simulink model "DisertatieVanca"  (R2021b)
settings: Solver=FixedStepAuto  StartTime=0.0  StopTime=10.0  RelTol=1e-3
undefined symbols (not defined in the file): DiscIntNeverNeededParam, Ion, Lithium, Ts, Ts_agent, Ts_speed
libraries: spsSeriesRLCBranchLib x10, spsDiodeLib x7, spsIGBTLib x6, mcbcontrolslib x3, simulink x3, spsVoltageMeasurementLib x3, spsThreePhaseVIMeasurementLib x3, spsCurrentMeasurementLib x2, spsBatteryLib x1, BatteryEstimators x1, spsIGBTDiodeLib x1, slpidlib x1
(part 2 of 2)

== system DisertatieVanca/Errors/BatterySafety ==
  SOC_Battery : Inport
  Voltage_Battery : Inport  Port=2
  Current_Battery : Inport  Port=3
  Power_Bat : Inport  Port=4
  Constant1 : Constant  Value=101  SampleTime=-1
  Constant2 : Constant  Value=-1  SampleTime=-1
  Constant3 : Constant  Value=900  SampleTime=-1
  Constant4 : Constant  Value=0  SampleTime=-1
  Constant6 : Constant  Value=0  SampleTime=-1
  Constant7 : Constant  Value=700  SampleTime=-1
  Constant8 : Constant  Value=0  SampleTime=-1
  Relational Operator1 : RelationalOperator  Operator=>  OutDataTypeStr=boolean  RndMeth=Simplest
  Relational Operator{2,4,6,8} (4 alike) : RelationalOperator  Operator=<  OutDataTypeStr=boolean  RndMeth=Simplest
  Relational Operator3 : RelationalOperator  Operator=>  OutDataTypeStr=boolean  RndMeth=Simplest
  Relational Operator7 : RelationalOperator  Operator=>  OutDataTypeStr=boolean  RndMeth=Simplest
  ErrBatterySOCMallfunctionLow : Outport
  ErrBatterySOCMallfunctionHigh : Outport  Port=2
  ErrBatteryVoltageLow : Outport  Port=3
  ErrBatteryVoltageHigh : Outport  Port=4
  ErrBatteryCurrentLow : Outport  Port=5
  ErrBatteryPowerLow : Outport  Port=6
  ErrBatteryPowerHigh : Outport  Port=7
  wires:
  Relational Operator2/1 -> ErrBatterySOCMallfunctionLow/1
  Relational Operator1/1 -> ErrBatterySOCMallfunctionHigh/1
  SOC_Battery/1 -> Relational Operator2/1, Relational Operator1/1
  Constant1/1 -> Relational Operator1/2
  Voltage_Battery/1 -> Relational Operator4/1, Relational Operator3/1
  Constant3/1 -> Relational Operator3/2
  Relational Operator3/1 -> ErrBatteryVoltageHigh/1
  Relational Operator4/1 -> ErrBatteryVoltageLow/1
  Constant6/1 -> Relational Operator6/1
  Relational Operator6/1 -> ErrBatteryCurrentLow/1
  Current_Battery/1 -> Relational Operator6/2
  Constant7/1 -> Relational Operator7/2
  Power_Bat/1 -> Relational Operator8/1, Relational Operator7/1
  Relational Operator7/1 -> ErrBatteryPowerHigh/1
  Relational Operator8/1 -> ErrBatteryPowerLow/1
  Constant2/1 -> Relational Operator2/2
  Constant4/1 -> Relational Operator4/2
  Constant8/1 -> Relational Operator8/2

== system DisertatieVanca/Errors/DCDCBoostSafety ==
  Vout : Inport
  Vin : Inport  Port=2
  iLref : Inport  Port=3
  Vref : Inport  Port=4
  S : Inport  Port=5
  Constant : Constant  Value=900
  Constant1 : Constant  Value=570  SampleTime=-1
  Constant2 : Constant  Value=480  SampleTime=-1
  Relational Operator : RelationalOperator  OutDataTypeStr=boolean  RndMeth=Simplest
  Relational Operator1 : RelationalOperator  Operator=>  OutDataTypeStr=boolean  RndMeth=Simplest
  Relational Operator2 : RelationalOperator  Operator=<  OutDataTypeStr=boolean  RndMeth=Simplest
  Terminator : Terminator
  Terminator1 : Terminator
  Terminator2 : Terminator
  ErrDCDCBoostOverVoltage : Outport
  ErrDCDCBoostInputVoltageLow : Outport  Port=2
  ErrDCDCBoostInputVoltageHigh : Outport  Port=3
  wires:
  Vout/1 -> Relational Operator/1
  Constant/1 -> Relational Operator/2
  Relational Operator/1 -> ErrDCDCBoostOverVoltage/1
  S/1 -> Terminator/1
  iLref/1 -> Terminator1/1
  Relational Operator1/1 -> ErrDCDCBoostInputVoltageHigh/1
  Constant1/1 -> Relational Operator1/2
  Relational Operator2/1 -> ErrDCDCBoostInputVoltageLow/1
  Vin/1 -> Relational Operator2/1, Relational Operator1/1
  Vref/1 -> Terminator2/1
  Constant2/1 -> Relational Operator2/2

== system DisertatieVanca/Errors/RectifierSafety ==
  VabcTriFazic : Inport
  CurrentValueRectifier : Inport  Port=2
  VoltageRectifier : Inport  Port=3
  MeanVoltageFromRec2 : Inport  Port=4
  MeanVoltageFromRec : Inport  Port=5
  Constant : Constant  Value=350  SampleTime=-1
  Constant1 : Constant  Value=-350  SampleTime=-1
  Constant2 : Constant  Value=700  SampleTime=-1
  Constant3 : Constant  Value=600  SampleTime=-1
  Constant4 : Constant  Value=450  SampleTime=-1
  Relational Operator : RelationalOperator  Operator=>  OutDataTypeStr=boolean  RndMeth=Simplest
  Relational Operator1 : RelationalOperator  Operator=<  OutDataTypeStr=boolean  RndMeth=Simplest
  Relational Operator2 : RelationalOperator  Operator=>  OutDataTypeStr=boolean  RndMeth=Simplest
  Relational Operator3 : RelationalOperator  Operator=>  OutDataTypeStr=boolean  RndMeth=Simplest
  Relational Operator4 : RelationalOperator  Operator=<  OutDataTypeStr=boolean  RndMeth=Simplest
  Terminator : Terminator
  Terminator1 : Terminator
  ErrTriFazicLow : Outport
  ErrTriFazicHigh : Outport  Port=2
  ErrTriFazicOverCurrent : Outport  Port=3
  ErrTriFazicLowVoltage : Outport  Port=4
  ErrTriFazicHighVoltage : Outport  Port=5
  wires:
  VabcTriFazic/1 -> Relational Operator1/1, Relational Operator/1
  Constant/1 -> Relational Operator/2
  Relational Operator/1 -> ErrTriFazicHigh/1
  Relational Operator1/1 -> ErrTriFazicLow/1
  Relational Operator2/1 -> ErrTriFazicOverCurrent/1
  Constant2/1 -> Relational Operator2/2
  CurrentValueRectifier/1 -> Relational Operator2/1
  Relational Operator3/1 -> ErrTriFazicHighVoltage/1
  Constant3/1 -> Relational Operator3/2
  Relational Operator4/1 -> ErrTriFazicLowVoltage/1
  VoltageRectifier/1 -> Relational Operator4/1, Relational Operator3/1
  MeanVoltageFromRec2/1 -> Terminator/1
  MeanVoltageFromRec/1 -> Terminator1/1
  Constant1/1 -> Relational Operator1/2
  Constant4/1 -> Relational Operator4/2

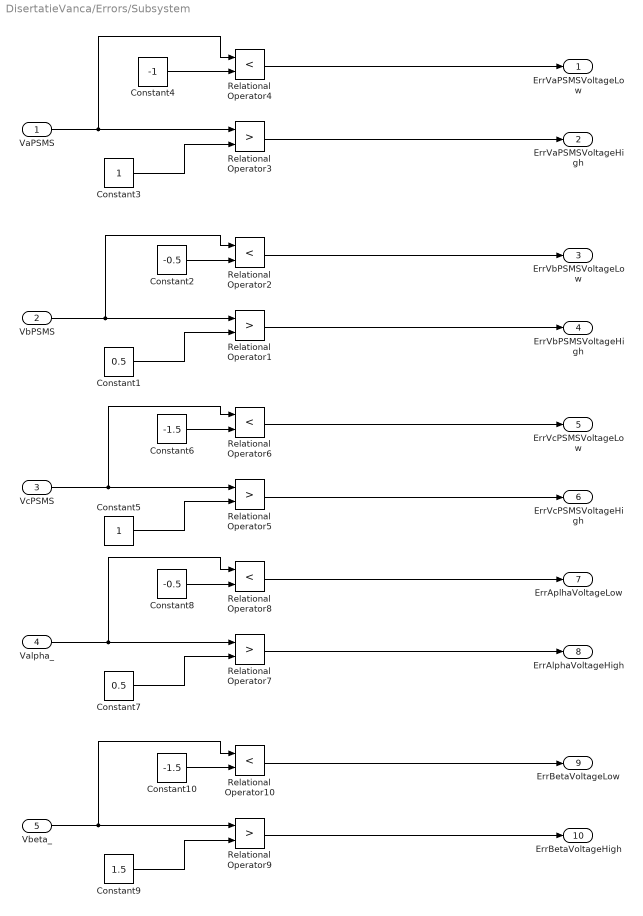
== system DisertatieVanca/Errors/Subsystem ==
  VaPSMS : Inport
  VbPSMS : Inport  Port=2
  VcPSMS : Inport  Port=3
  Valpha_ : Inport  Port=4
  Vbeta_ : Inport  Port=5
  Constant1 : Constant  Value=0.5  SampleTime=-1
  Constant10 : Constant  Value=-1.5  SampleTime=-1
  Constant2 : Constant  Value=-0.5  SampleTime=-1
  Constant3 : Constant  SampleTime=-1
  Constant4 : Constant  Value=-1  SampleTime=-1
  Constant5 : Constant  SampleTime=-1
  Constant6 : Constant  Value=-1.5  SampleTime=-1
  Constant7 : Constant  Value=0.5  SampleTime=-1
  Constant8 : Constant  Value=-0.5  SampleTime=-1
  Constant9 : Constant  Value=1.5  SampleTime=-1
  Relational Operator{1,3,5,7,9} (5 alike) : RelationalOperator  Operator=>  OutDataTypeStr=boolean  RndMeth=Simplest
  Relational Operator{2,4,6,8,10} (5 alike) : RelationalOperator  Operator=<  OutDataTypeStr=boolean  RndMeth=Simplest
  ErrVaPSMSVoltageLow : Outport
  ErrVaPSMSVoltageHigh : Outport  Port=2
  ErrVbPSMSVoltageLow : Outport  Port=3
  ErrVbPSMSVoltageHigh : Outport  Port=4
  ErrVcPSMSVoltageLow : Outport  Port=5
  ErrVcPSMSVoltageHigh : Outport  Port=6
  ErrAplhaVoltageLow : Outport  Port=7
  ErrAlphaVoltageHigh : Outport  Port=8
  ErrBetaVoltageLow : Outport  Port=9
  ErrBetaVoltageHigh : Outport  Port=10
  wires:
  Relational Operator3/1 -> ErrVaPSMSVoltageHigh/1
  Relational Operator4/1 -> ErrVaPSMSVoltageLow/1
  Constant3/1 -> Relational Operator3/2
  VaPSMS/1 -> Relational Operator4/1, Relational Operator3/1
  Relational Operator1/1 -> ErrVbPSMSVoltageHigh/1
  Relational Operator2/1 -> ErrVbPSMSVoltageLow/1
  Constant1/1 -> Relational Operator1/2
  VbPSMS/1 -> Relational Operator2/1, Relational Operator1/1
  Relational Operator5/1 -> ErrVcPSMSVoltageHigh/1
  Relational Operator6/1 -> ErrVcPSMSVoltageLow/1
  Constant5/1 -> Relational Operator5/2
  VcPSMS/1 -> Relational Operator6/1, Relational Operator5/1
  Relational Operator7/1 -> ErrAlphaVoltageHigh/1
  Relational Operator8/1 -> ErrAplhaVoltageLow/1
  Constant7/1 -> Relational Operator7/2
  Valpha_/1 -> Relational Operator8/1, Relational Operator7/1
  Relational Operator9/1 -> ErrBetaVoltageHigh/1
  Relational Operator10/1 -> ErrBetaVoltageLow/1
  Constant9/1 -> Relational Operator9/2
  Vbeta_/1 -> Relational Operator10/1, Relational Operator9/1
  Constant4/1 -> Relational Operator4/2
  Constant2/1 -> Relational Operator2/2
  Constant6/1 -> Relational Operator6/2
  Constant8/1 -> Relational Operator8/2
  Constant10/1 -> Relational Operator10/2

== system DisertatieVanca/Errors/Subsystem1 ==
  IdRef : Inport
  IqRef : Inport  Port=2
  Id_ : Inport  Port=3
  Iq_ : Inport  Port=4
  speed_fb : Inport  Port=5
  speed_ref : Inport  Port=6
  Constant1 : Constant  Value=-1  SampleTime=-1
  Constant10 : Constant  SampleTime=-1
  Constant2 : Constant  SampleTime=-1
  Constant3 : Constant  Value=-1.5  SampleTime=-1
  Constant4 : Constant  Value=1.5  SampleTime=-1
  Constant9 : Constant  Value=3  SampleTime=-1
  Relational Operator1 : RelationalOperator  Operator=<  OutDataTypeStr=boolean  RndMeth=Simplest
  Relational Operator10 : RelationalOperator  Operator=<  OutDataTypeStr=boolean  RndMeth=Simplest
  Relational Operator2 : RelationalOperator  Operator=>  OutDataTypeStr=boolean  RndMeth=Simplest
  Relational Operator3 : RelationalOperator  Operator=<  OutDataTypeStr=boolean  RndMeth=Simplest
  Relational Operator4 : RelationalOperator  Operator=>  OutDataTypeStr=boolean  RndMeth=Simplest
  Relational Operator9 : RelationalOperator  Operator=>  OutDataTypeStr=boolean  RndMeth=Simplest
  Terminator : Terminator
  Terminator1 : Terminator
  Terminator2 : Terminator
  ErrSpeedVoltageLow : Outport
  ErrSpeedVoltageHigh : Outport  Port=2
  ErrIdLow : Outport  Port=3
  ErrIdHigh : Outport  Port=4
  ErrIqLow : Outport  Port=5
  ErrIqHigh : Outport  Port=6
  wires:
  IdRef/1 -> Terminator/1
  IqRef/1 -> Terminator1/1
  speed_ref/1 -> Terminator2/1
  Relational Operator10/1 -> ErrSpeedVoltageLow/1
  Constant9/1 -> Relational Operator9/2
  speed_fb/1 -> Relational Operator10/1, Relational Operator9/1
  Relational Operator9/1 -> ErrSpeedVoltageHigh/1
  Relational Operator1/1 -> ErrIdLow/1
  Constant2/1 -> Relational Operator2/2
  Id_/1 -> Relational Operator1/1, Relational Operator2/1
  Relational Operator2/1 -> ErrIdHigh/1
  Relational Operator3/1 -> ErrIqLow/1
  Constant4/1 -> Relational Operator4/2
  Iq_/1 -> Relational Operator3/1, Relational Operator4/1
  Relational Operator4/1 -> ErrIqHigh/1
  Constant10/1 -> Relational Operator10/2
  Constant1/1 -> Relational Operator1/2
  Constant3/1 -> Relational Operator3/2

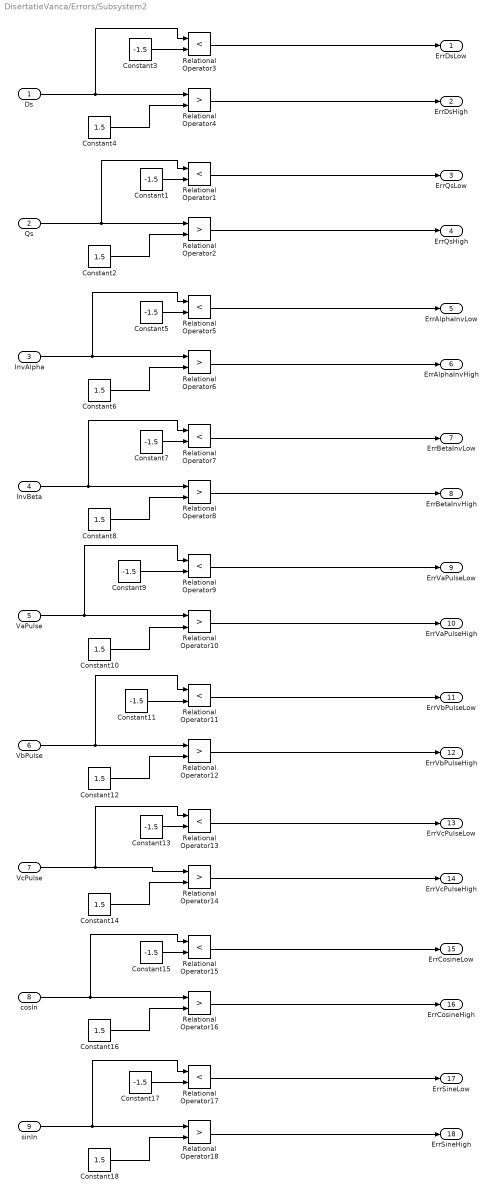
== system DisertatieVanca/Errors/Subsystem2 ==
  Ds : Inport
  Qs : Inport  Port=2
  InvAlpha : Inport  Port=3
  InvBeta : Inport  Port=4
  VaPulse : Inport  Port=5
  VbPulse : Inport  Port=6
  VcPulse : Inport  Port=7
  cosIn : Inport  Port=8
  sinIn : Inport  Port=9
  Constant{1,3,5,7,9,11,13,15,17} (9 alike) : Constant  Value=-1.5  SampleTime=-1
  Constant{2,4,6,8,10,12,14,16,18} (9 alike) : Constant  Value=1.5  SampleTime=-1
  Relational Operator{1,3,5,7,9,11,13,15,17} (9 alike) : RelationalOperator  Operator=<  OutDataTypeStr=boolean  RndMeth=Simplest
  Relational Operator{2,4,6,8,10,12,14,16,18} (9 alike) : RelationalOperator  Operator=>  OutDataTypeStr=boolean  RndMeth=Simplest
  ErrDsLow : Outport
  ErrDsHigh : Outport  Port=2
  ErrQsLow : Outport  Port=3
  ErrQsHigh : Outport  Port=4
  ErrAlphaInvLow : Outport  Port=5
  ErrAlphaInvHigh : Outport  Port=6
  ErrBetaInvLow : Outport  Port=7
  ErrBetaInvHigh : Outport  Port=8
  ErrVaPulseLow : Outport  Port=9
  ErrVaPulseHigh : Outport  Port=10
  ErrVbPulseLow : Outport  Port=11
  ErrVbPulseHigh : Outport  Port=12
  ErrVcPulseLow : Outport  Port=13
  ErrVcPulseHigh : Outport  Port=14
  ErrCosineLow : Outport  Port=15
  ErrCosineHigh : Outport  Port=16
  ErrSineLow : Outport  Port=17
  ErrSineHigh : Outport  Port=18
  wires:
  Relational Operator3/1 -> ErrDsLow/1
  Relational Operator4/1 -> ErrDsHigh/1
  Constant4/1 -> Relational Operator4/2
  Ds/1 -> Relational Operator3/1, Relational Operator4/1
  Relational Operator1/1 -> ErrQsLow/1
  Relational Operator2/1 -> ErrQsHigh/1
  Constant2/1 -> Relational Operator2/2
  Qs/1 -> Relational Operator1/1, Relational Operator2/1
  Relational Operator6/1 -> ErrAlphaInvHigh/1
  Relational Operator5/1 -> ErrAlphaInvLow/1
  InvAlpha/1 -> Relational Operator5/1, Relational Operator6/1
  Constant6/1 -> Relational Operator6/2
  Relational Operator8/1 -> ErrBetaInvHigh/1
  Relational Operator7/1 -> ErrBetaInvLow/1
  InvBeta/1 -> Relational Operator7/1, Relational Operator8/1
  Constant8/1 -> Relational Operator8/2
  VaPulse/1 -> Relational Operator9/1, Relational Operator10/1
  Relational Operator10/1 -> ErrVaPulseHigh/1
  Constant10/1 -> Relational Operator10/2
  Relational Operator9/1 -> ErrVaPulseLow/1
  VbPulse/1 -> Relational Operator11/1, Relational Operator12/1
  Relational Operator12/1 -> ErrVbPulseHigh/1
  Constant12/1 -> Relational Operator12/2
  Relational Operator11/1 -> ErrVbPulseLow/1
  VcPulse/1 -> Relational Operator13/1, Relational Operator14/1
  Relational Operator14/1 -> ErrVcPulseHigh/1
  Constant14/1 -> Relational Operator14/2
  Relational Operator13/1 -> ErrVcPulseLow/1
  cosIn/1 -> Relational Operator15/1, Relational Operator16/1
  Relational Operator16/1 -> ErrCosineHigh/1
  Constant16/1 -> Relational Operator16/2
  Relational Operator15/1 -> ErrCosineLow/1
  sinIn/1 -> Relational Operator17/1, Relational Operator18/1
  Relational Operator18/1 -> ErrSineHigh/1
  Constant18/1 -> Relational Operator18/2
  Relational Operator17/1 -> ErrSineLow/1
  Constant3/1 -> Relational Operator3/2
  Constant1/1 -> Relational Operator1/2
  Constant5/1 -> Relational Operator5/2
  Constant7/1 -> Relational Operator7/2
  Constant9/1 -> Relational Operator9/2
  Constant11/1 -> Relational Operator11/2
  Constant13/1 -> Relational Operator13/2
  Constant15/1 -> Relational Operator15/2
  Constant17/1 -> Relational Operator17/2

== system DisertatieVanca/Errors Clasification/High Severity ==
  ErrTriFazicOverCurrent : Inport
  ErrBatterySOCMallfunctionLow : Inport  Port=2
  ErrBatterySOCMallfunctionHigh : Inport  Port=3
  ErrDCDCBoostOverVoltage : Inport  Port=4
  ErrDCDCBoostInputVoltageHigh : Inport  Port=5
  Bus Creator : BusCreator  Inputs=5
  Constant{,1..4} (5 alike) : Constant  Value=0  SampleTime=-1
  Relational Operator{,1..4} (5 alike) : RelationalOperator  Operator=>  OutDataTypeStr=boolean  RndMeth=Simplest
  High_Severity : Outport
  wires:
  Constant/1 -> Relational Operator/2
  ErrBatterySOCMallfunctionLow/1 -> Relational Operator1/1
  Constant1/1 -> Relational Operator1/2
  ErrBatterySOCMallfunctionHigh/1 -> Relational Operator2/1
  Constant2/1 -> Relational Operator2/2
  ErrDCDCBoostOverVoltage/1 -> Relational Operator3/1
  Constant3/1 -> Relational Operator3/2
  ErrDCDCBoostInputVoltageHigh/1 -> Relational Operator4/1
  Constant4/1 -> Relational Operator4/2
  ErrTriFazicOverCurrent/1 -> Relational Operator/1
  Relational Operator2/1 -> Bus Creator/3
  Relational Operator1/1 -> Bus Creator/2
  Relational Operator/1 -> Bus Creator/1
  Relational Operator3/1 -> Bus Creator/4
  Relational Operator4/1 -> Bus Creator/5
  Bus Creator/1 -> High_Severity/1

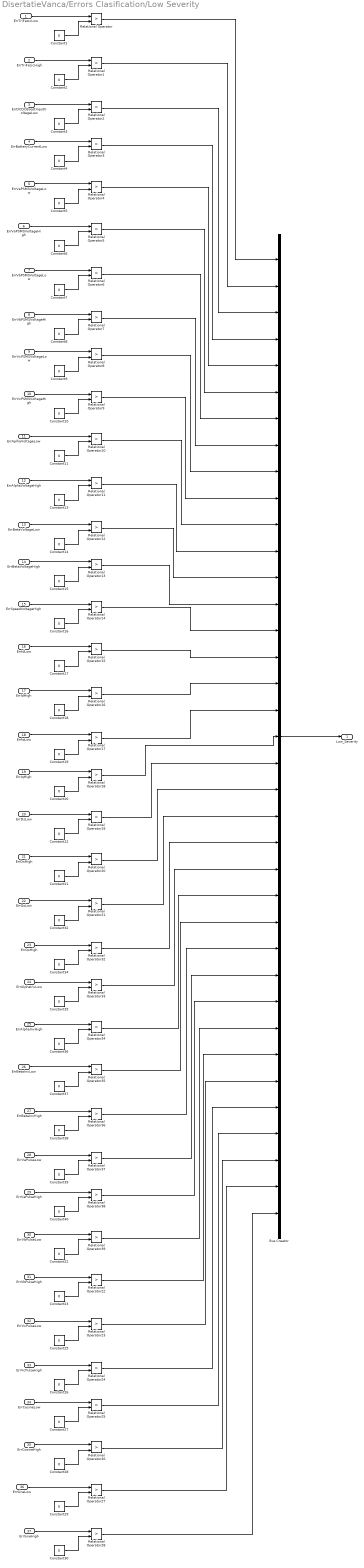
== system DisertatieVanca/Errors Clasification/Low Severity ==
  ErrTriFazicLow : Inport
  ErrTriFazicHigh : Inport  Port=2
  ErrDCDCBoostInputVoltageLow : Inport  Port=3
  ErrBatteryCurrentLow : Inport  Port=4
  ErrVaPSMSVoltageLow : Inport  Port=5
  ErrVaPSMSVoltageHigh : Inport  Port=6
  ErrVbPSMSVoltageLow : Inport  Port=7
  ErrVbPSMSVoltageHigh : Inport  Port=8
  ErrVcPSMSVoltageLow : Inport  Port=9
  ErrVcPSMSVoltageHigh : Inport  Port=10
  ErrAplhaVoltageLow : Inport  Port=11
  ErrAlphaVoltageHigh : Inport  Port=12
  ErrBetaVoltageLow : Inport  Port=13
  ErrBetaVoltageHigh : Inport  Port=14
  ErrSpeedVoltageHigh : Inport  Port=15
  ErrIdLow : Inport  Port=16
  ErrIdHigh : Inport  Port=17
  ErrIqLow : Inport  Port=18
  ErrIqHigh : Inport  Port=19
  ErrDsLow : Inport  Port=20
  ErrDsHigh : Inport  Port=21
  ErrQsLow : Inport  Port=22
  ErrQsHigh : Inport  Port=23
  ErrAlphaInvLow : Inport  Port=24
  ErrAlphaInvHigh : Inport  Port=25
  ErrBetaInvLow : Inport  Port=26
  ErrBetaInvHigh : Inport  Port=27
  ErrVaPulseLow : Inport  Port=28
  ErrVaPulseHigh : Inport  Port=29
  ErrVbPulseLow : Inport  Port=30
  ErrVbPulseHigh : Inport  Port=31
  ErrVcPulseLow : Inport  Port=32
  ErrVcPulseHigh : Inport  Port=33
  ErrCosineLow : Inport  Port=34
  ErrCosineHigh : Inport  Port=35
  ErrSineLow : Inport  Port=36
  ErrSineHigh : Inport  Port=37
  Bus Creator : BusCreator  Inputs=37
  Constant{1..23,25..30,32,34..40} (37 alike) : Constant  Value=0  SampleTime=-1
  Relational Operator{,1..28,32..39} (37 alike) : RelationalOperator  Operator=>  OutDataTypeStr=boolean  RndMeth=Simplest
  Low_Severity : Outport
  wires:
  Constant1/1 -> Relational Operator/2
  ErrTriFazicLow/1 -> Relational Operator/1
  Constant2/1 -> Relational Operator1/2
  ErrTriFazicHigh/1 -> Relational Operator1/1
  Constant3/1 -> Relational Operator2/2
  ErrDCDCBoostInputVoltageLow/1 -> Relational Operator2/1
  Constant4/1 -> Relational Operator3/2
  ErrBatteryCurrentLow/1 -> Relational Operator3/1
  Constant5/1 -> Relational Operator4/2
  ErrVaPSMSVoltageLow/1 -> Relational Operator4/1
  ErrVcPSMSVoltageLow/1 -> Relational Operator8/1
  ErrVaPSMSVoltageHigh/1 -> Relational Operator5/1
  ErrVbPSMSVoltageLow/1 -> Relational Operator6/1
  Constant8/1 -> Relational Operator7/2
  ErrVbPSMSVoltageHigh/1 -> Relational Operator7/1
  ErrVcPSMSVoltageHigh/1 -> Relational Operator9/1
  Constant6/1 -> Relational Operator5/2
  Constant7/1 -> Relational Operator6/2
  Constant10/1 -> Relational Operator9/2
  Constant9/1 -> Relational Operator8/2
  ErrDsLow/1 -> Relational Operator19/1
  ErrBetaVoltageHigh/1 -> Relational Operator13/1
  ErrAplhaVoltageLow/1 -> Relational Operator10/1
  ErrAlphaVoltageHigh/1 -> Relational Operator11/1
  Constant11/1 -> Relational Operator10/2
  ErrSpeedVoltageHigh/1 -> Relational Operator14/1
  Constant15/1 -> Relational Operator13/2
  Constant14/1 -> Relational Operator12/2
  ErrIqLow/1 -> Relational Operator17/1
  ErrIdLow/1 -> Relational Operator15/1
  ErrBetaVoltageLow/1 -> Relational Operator12/1
  Constant20/1 -> Relational Operator18/2
  Constant17/1 -> Relational Operator15/2
  Constant19/1 -> Relational Operator17/2
  Constant18/1 -> Relational Operator16/2
  ErrIqHigh/1 -> Relational Operator18/1
  Constant13/1 -> Relational Operator11/2
  ErrIdHigh/1 -> Relational Operator16/1
  Constant16/1 -> Relational Operator14/2
  Constant12/1 -> Relational Operator19/2
  ErrAlphaInvLow/1 -> Relational Operator33/1
  ErrDsHigh/1 -> Relational Operator20/1
  ErrCosineLow/1 -> Relational Operator25/1
  ErrQsLow/1 -> Relational Operator21/1
  ErrVbPulseHigh/1 -> Relational Operator22/1
  ErrSineHigh/1 -> Relational Operator28/1
  Constant21/1 -> Relational Operator20/2
  ErrAlphaInvHigh/1 -> Relational Operator34/1
  ErrCosineHigh/1 -> Relational Operator26/1
  Constant34/1 -> Relational Operator32/2
  ErrVaPulseLow/1 -> Relational Operator37/1
  ErrSineLow/1 -> Relational Operator27/1
  ErrQsHigh/1 -> Relational Operator32/1
  ErrVcPulseHigh/1 -> Relational Operator24/1
  Constant40/1 -> Relational Operator38/2
  Constant39/1 -> Relational Operator37/2
  Constant37/1 -> Relational Operator35/2
  Constant38/1 -> Relational Operator36/2
  Constant32/1 -> Relational Operator21/2
  Constant30/1 -> Relational Operator28/2
  Constant25/1 -> Relational Operator23/2
  Constant22/1 -> Relational Operator39/2
  Constant27/1 -> Relational Operator25/2
  Constant29/1 -> Relational Operator27/2
  Constant23/1 -> Relational Operator22/2
  ErrVbPulseLow/1 -> Relational Operator39/1
  ErrVaPulseHigh/1 -> Relational Operator38/1
  ErrBetaInvHigh/1 -> Relational Operator36/1
  Constant36/1 -> Relational Operator34/2
  Constant26/1 -> Relational Operator24/2
  Constant35/1 -> Relational Operator33/2
  ErrVcPulseLow/1 -> Relational Operator23/1
  Constant28/1 -> Relational Operator26/2
  ErrBetaInvLow/1 -> Relational Operator35/1
  Relational Operator/1 -> Bus Creator/1
  Relational Operator1/1 -> Bus Creator/2
  Relational Operator2/1 -> Bus Creator/3
  Relational Operator3/1 -> Bus Creator/4
  Relational Operator4/1 -> Bus Creator/5
  Relational Operator5/1 -> Bus Creator/6
  Relational Operator6/1 -> Bus Creator/7
  Relational Operator7/1 -> Bus Creator/8
  Relational Operator8/1 -> Bus Creator/9
  Relational Operator9/1 -> Bus Creator/10
  Relational Operator10/1 -> Bus Creator/11
  Relational Operator11/1 -> Bus Creator/12
  Relational Operator12/1 -> Bus Creator/13
  Relational Operator13/1 -> Bus Creator/14
  Relational Operator14/1 -> Bus Creator/15
  Relational Operator15/1 -> Bus Creator/16
  Relational Operator16/1 -> Bus Creator/17
  Relational Operator17/1 -> Bus Creator/18
  Relational Operator18/1 -> Bus Creator/19
  Relational Operator19/1 -> Bus Creator/20
  Relational Operator20/1 -> Bus Creator/21
  Relational Operator21/1 -> Bus Creator/22
  Relational Operator32/1 -> Bus Creator/23
  Relational Operator33/1 -> Bus Creator/24
  Relational Operator34/1 -> Bus Creator/25
  Relational Operator35/1 -> Bus Creator/26
  Relational Operator36/1 -> Bus Creator/27
  Relational Operator37/1 -> Bus Creator/28
  Relational Operator38/1 -> Bus Creator/29
  Relational Operator39/1 -> Bus Creator/30
  Relational Operator22/1 -> Bus Creator/31
  Relational Operator23/1 -> Bus Creator/32
  Relational Operator24/1 -> Bus Creator/33
  Relational Operator25/1 -> Bus Creator/34
  Relational Operator26/1 -> Bus Creator/35
  Relational Operator27/1 -> Bus Creator/36
  Relational Operator28/1 -> Bus Creator/37
  Bus Creator/1 -> Low_Severity/1

== system DisertatieVanca/Errors Clasification/Medium Severity ==
  ErrTriFazicLowVoltage : Inport
  ErrTriFazicHighVoltage : Inport  Port=2
  ErrBatteryVoltageLow : Inport  Port=3
  ErrBatteryVoltageHigh : Inport  Port=4
  ErrBatteryPowerLow : Inport  Port=5
  ErrBatteryPowerHigh : Inport  Port=6
  ErrSpeedVoltageLow : Inport  Port=7
  Bus Creator : BusCreator  Inputs=7
  Constant{1..7} (7 alike) : Constant  Value=0  SampleTime=-1
  Relational Operator{,1..6} (7 alike) : RelationalOperator  Operator=>  OutDataTypeStr=boolean  RndMeth=Simplest
  Medium_Severity : Outport
  wires:
  ErrTriFazicLowVoltage/1 -> Relational Operator/1
  Constant1/1 -> Relational Operator/2
  Constant2/1 -> Relational Operator1/2
  ErrTriFazicHighVoltage/1 -> Relational Operator1/1
  Constant3/1 -> Relational Operator2/2
  ErrBatteryVoltageLow/1 -> Relational Operator2/1
  Constant4/1 -> Relational Operator3/2
  ErrBatteryVoltageHigh/1 -> Relational Operator3/1
  Constant5/1 -> Relational Operator4/2
  ErrBatteryPowerLow/1 -> Relational Operator4/1
  Constant6/1 -> Relational Operator5/2
  ErrBatteryPowerHigh/1 -> Relational Operator5/1
  Constant7/1 -> Relational Operator6/2
  ErrSpeedVoltageLow/1 -> Relational Operator6/1
  Relational Operator3/1 -> Bus Creator/4
  Relational Operator2/1 -> Bus Creator/3
  Relational Operator1/1 -> Bus Creator/2
  Relational Operator/1 -> Bus Creator/1
  Relational Operator4/1 -> Bus Creator/5
  Relational Operator5/1 -> Bus Creator/6
  Relational Operator6/1 -> Bus Creator/7
  Bus Creator/1 -> Medium_Severity/1

== system DisertatieVanca/Reinforcement Learning/IsDone ==
  Iq_ref : Inport
  Compare To Constant2 : simulink/Logic and Bit Operations/Compare To Constant  relop=>=  const=0.3  OutDataTypeStr=boolean
  Compare To Constant3 : simulink/Logic and Bit Operations/Compare To Constant  relop=>=  const=1  OutDataTypeStr=boolean
  Digital Clock : DigitalClock  SampleTime=Ts_agent
  OR1 : Logic  IconShape=distinctive  AllPortsSameDT=off  OutDataTypeStr=boolean
  Product : Product
  TrainFlag : Constant  OutDataTypeStr=double
  stop : Outport
  wires:
  TrainFlag/1 -> Product/2
  Product/1 -> stop/1
  Digital Clock/1 -> Compare To Constant2/1
  OR1/1 -> Product/1
  Compare To Constant3/1 -> OR1/1
  Iq_ref/1 -> Compare To Constant3/1
  Compare To Constant2/1 -> OR1/2

== system DisertatieVanca/Reinforcement Learning/Observations ==
  speed ref : Inport
  speed fb : Inport  Port=2
  id err : Inport  Port=3
  id : Inport  Port=4
  iq err : Inport  Port=5
  iq : Inport  Port=6
  Discrete-Time Integrator : DiscreteIntegrator  SampleTime=-1  ICPrevOutput=DiscIntNeverNeededParam  ICPrevScaledInput=DiscIntNeverNeededParam
  Discrete-Time Integrator1 : DiscreteIntegrator  SampleTime=-1  ICPrevOutput=DiscIntNeverNeededParam  ICPrevScaledInput=DiscIntNeverNeededParam
  Mux1 : Mux  Inputs=8
  observations : Outport  VectorParamsAs1DForOutWhenUnconnected=off
  wires:
  id err/1 -> Discrete-Time Integrator/1, Mux1/5
  Discrete-Time Integrator/1 -> Mux1/6
  iq err/1 -> Discrete-Time Integrator1/1, Mux1/7
  Discrete-Time Integrator1/1 -> Mux1/8
  Mux1/1 -> observations/1
  iq/1 -> Mux1/4
  id/1 -> Mux1/3
  speed fb/1 -> Mux1/2
  speed ref/1 -> Mux1/1

== system DisertatieVanca/Reinforcement Learning/Reward ==
  id error : Inport
  iq error : Inport  Port=2
  done : Inport  Port=3
  action : Inport  Port=4
  " r(1,2,3,4,5)" : Scope  NumInputPorts=5
  Add1 : Sum  Inputs=+++++
  Demux : Demux  Outputs=2
  Gain : Gain  Gain=-5
  Gain1 : Gain  Gain=-0.1
  Gain2 : Gain  Gain=-100
  Gain3 : Gain  Gain=-5
  Gain5 : Gain  Gain=-0.1
  Reward : Scope
  Square{,1..3} (4 alike) : Math  Operator=square  SaturateOnIntegerOverflow=on
  reward : Outport  VectorParamsAs1DForOutWhenUnconnected=off
  wires:
  done/1 -> Gain2/1
  Gain2/1 -> " r(1,2,3,4,5)"/5, Add1/5  "r5"
  iq error/1 -> Square2/1
  id error/1 -> Square1/1
  Gain3/1 -> Add1/2, " r(1,2,3,4,5)"/2  "r2"
  Gain/1 -> Add1/1, " r(1,2,3,4,5)"/1  "r1"
  Gain5/1 -> Add1/4, " r(1,2,3,4,5)"/4  "r4"
  Add1/1 -> reward/1, Reward/1
  action/1 -> Demux/1
  Square3/1 -> Gain5/1
  Demux/2 -> Square3/1
  Gain1/1 -> Add1/3, " r(1,2,3,4,5)"/3  "r3"
  Square/1 -> Gain1/1
  Demux/1 -> Square/1
  Square2/1 -> Gain3/1
  Square1/1 -> Gain/1

== matlab function DisertatieVanca/DCC_Boost/MATLAB Function ==
  settings: updateMethod=DISCRETE
  data: iL input; S output; Vin input; Vout input; iL_ref input; wf input
function S = MPC_Boost(iL,Vin,Vout,iL_ref,wf)
Ts=10e-6;
L=0.003;
RL=1.5;
States=[1;0];
g_op=1e6;
n_op=1;
persistent S_old;
if isempty(S_old)
    S_old=0;
end
for n=1:2
    iL_k1=(Ts/L)*(Vin-iL*RL-Vout*(1-States(n)))+iL;
    g_sw=abs(States(n)-S_old);
    g_iL=abs(iL_ref-iL_k1); %cost function
    g=g_iL+g_sw*wf;
    if(g<g_op)
        n_op=n;
        g_op=g;
    end
end
S=States(n_op);
S_old=S;
